simulink model "target_gen_logic_test"  (R2018b)
settings: Solver=VariableStepAuto  StartTime=0.0  StopTime=10.0  RelTol=1e-3
libraries: target_gen_logic_lib x1
settings Model: Creator=Taylor  LastModifiedBy=Taylor

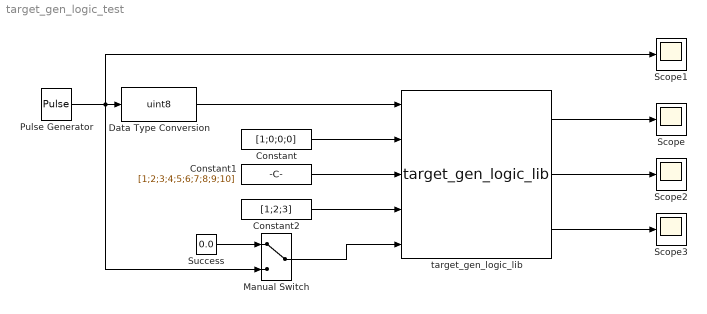
== system target_gen_logic_test ==
  Constant : Constant  Value=[1;0;0;0]
  Constant1 : Constant  Value=[1;2;3;4;5;6;7;8;9;10]
  Constant2 : Constant  Value=[1;2;3]
  Data Type Conversion : DataTypeConversion  OutDataTypeStr=uint8
  Manual Switch : ManualSwitch
  Pulse Generator : DiscretePulseGenerator  PulseType=Time based  Amplitude=8  Period=5  PulseWidth=25  PhaseDelay=1
  Scope{,1..3} (4 alike) : Scope
  Success : Constant  Value=0.0
  target_gen_logic_lib : target_gen_logic_lib/target_gen_logic_lib  SystemSampleTime=-1
  wires:
  Data Type Conversion/1 -> target_gen_logic_lib/1
  Constant/1 -> target_gen_logic_lib/2
  Constant1/1 -> target_gen_logic_lib/3
  Constant2/1 -> target_gen_logic_lib/4
  target_gen_logic_lib/1 -> Scope/1
  target_gen_logic_lib/2 -> Scope2/1
  target_gen_logic_lib/3 -> Scope3/1
  Pulse Generator/1 -> Manual Switch/2, Scope1/1, Data Type Conversion/1
  Success/1 -> Manual Switch/1
  Manual Switch/1 -> target_gen_logic_lib/5
